simulink model "controllo_SS2023b"  (R2023b)
settings: Solver=VariableStepAuto  StartTime=0.0  StopTime=y1(end,1)  RelTol=1e-3
values from neighbouring files (symbols this model uses):
  A_ob = A - L_kf*C    [LQ_KF.m]    (also in LQ_KF_version1.m; LQ_KF_version2.m; LQ_Luenberger.m = A - L*C; LQ_prova.m)
  B_ob = [ B - L_kf*D, L_kf]    [LQ_KF.m]    (also in LQ_KF_version1.m; LQ_KF_version2.m; LQ_Luenberger.m = [ B - L*D, L]; LQ_prova.m)
  C_ob = eye(n)    [LQ_KF.m]    (also in LQ_KF_version1.m; LQ_KF_version2.m; LQ_Luenberger.m; LQ_prova.m)
  D_ob = zeros(n, m+p)    [LQ_KF.m]    (also in LQ_KF_version1.m; LQ_KF_version2.m; LQ_Luenberger.m; LQ_prova.m)
  Ken_eta = K(:, 4)    [LQ_KF.m]    (also in LQ_KF_version1.m; LQ_KF_version2.m = Ken(:, n+1:end); LQ_Luenberger.m; LQ_prova.m = Ken(:, n+1:end))
  Ken_x = K(:, 1:3)    [LQ_KF.m]    (also in LQ_KF_version1.m; LQ_KF_version2.m = Ken(:, 1:n); LQ_Luenberger.m; LQ_prova.m = Ken(:, 1:n))
undefined symbols (not defined in the file or in its folder): Lc, Rtot, x1_eq0, x2_eq0, x3_eq0
libraries: simulink x1
settings Model: Creator=Pronto all'uso  LastModifiedBy=Pronto all'uso

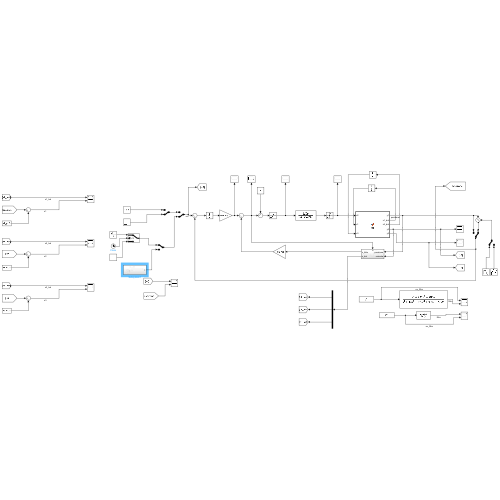
[thumbnail: Simulink's stored preview of the top-level diagram]
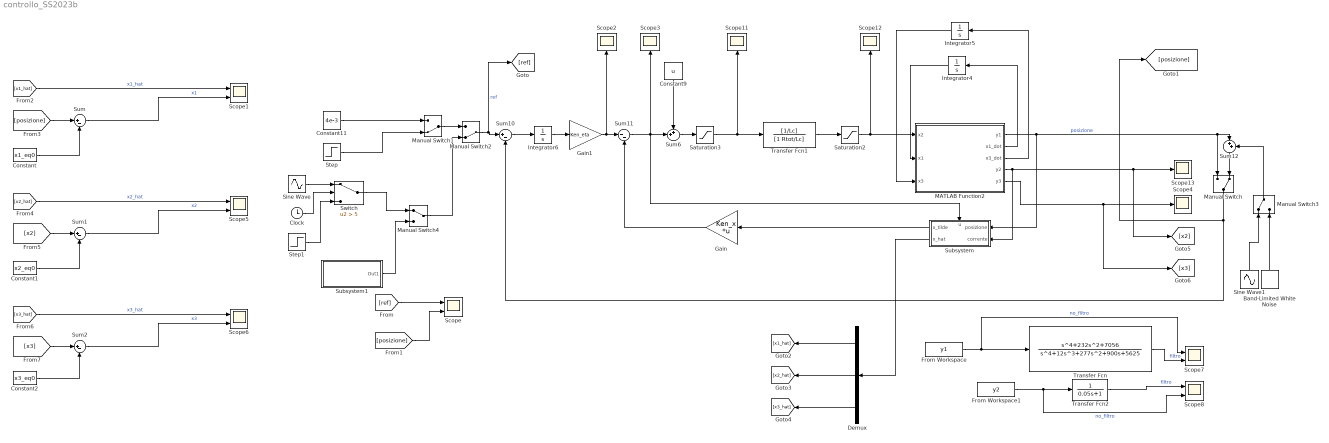
== system controllo_SS2023b ==
  Band-Limited White Noise : simulink/Sources/Band-Limited White Noise  Cov=[8.9934e-8*0.002]  Ts=0.002  seed=[23341]
  Clock : Clock
  Constant : Constant  Value=x1_eq0
  Constant1 : Constant  Value=x2_eq0
  Constant11 : Constant  Value=4e-3
  Constant2 : Constant  Value=x3_eq0
  Constant9 : Constant  Value=u
  Demux : Demux  Outputs=3
  From Workspace : FromWorkspace  VariableName=y1
  From Workspace1 : FromWorkspace  VariableName=y2
  Gain : Gain  Gain=Ken_x  Multiplication=Matrix(K*u) (u vector)
  Gain1 : Gain  Gain=Ken_eta
  Integrator4 : Integrator
  Integrator5 : Integrator
  Integrator6 : Integrator
  MATLAB Function2 : MATLAB Function  TreatAsAtomicUnit=on
  Manual Switch : ManualSwitch  CurrentSetting=0
  Manual Switch1 : ManualSwitch  CurrentSetting=0
  Manual Switch2 : ManualSwitch  CurrentSetting=0
  Manual Switch3 : ManualSwitch
  Manual Switch4 : ManualSwitch
  Saturation2 : Saturate  UpperLimit=3  LowerLimit=0
  Saturation3 : Saturate  UpperLimit=24  LowerLimit=0
  Scope{,1,5..8} (6 alike) : Scope  NumInputPorts=2
  Scope{2..4,11..13} (6 alike) : Scope
  Sine Wave : Sin  Amplitude=0.0005  Bias=0.004  SampleTime=0
  Sine Wave1 : Sin  Amplitude=0.00001  Frequency=50  SampleTime=0.002
  Step : Step  Time=2  After=0.003  SampleTime=0.002
  Step1 : Step  Time=3  After=0.004  SampleTime=0
  Subsystem : Subsystem
      settings: PortSchema="{\"entries\":[{\"content\":{\"sides\":[{\"content\":{\"connectorIds\":[\"In1\",\"In2\"]},\"type\":\"ConnectorPlacement.EquallySpacedRectSide\",\"uuid\":\"698df1f3-7755-43c0-a5fb-5bdaf8e9b8ef\"},{\"content\":{\"connectorIds\":[\"Out1\",\"Out2\"],\"side\":\"RIGHT\"},\"type\":\"ConnectorPlacement.EquallySpacedRectSide\",\"uuid\":\"f0019f40-b27c-431f-9c37-04fd54da4bcb\"},{\"content\":{\"connectorIds\":[\"In3\"],\"side\":\"TOP\"},\"type\":\"ConnectorPlacement.EquallySpacedRectSide\",\"uuid\":\"7983fe5a-f7de-4e42-be2b-50e780fdde63\"}]},\"type\":\"ConnectorPlacement.EquallySpacedConnector\",\"uuid\":\"65d76084-d1f3-463d-b10f-a9e5fd5bbc83\"}],\"packageUris\":[\"http://schema.mathworks.com/mf0/Connector/R2020b\"],\"version\":\"1.0\"}"
  Subsystem1 : Subsystem
  Sum{,1..2,10} (4 alike) : Sum  Inputs=|+-
  Sum11 : Sum  Inputs=|--
  Sum12 : Sum  Inputs=|++
  Sum6 : Sum  Inputs=++|
  Switch : Switch  Criteria=u2 > Threshold  Threshold=5  SaturateOnIntegerOverflow=off  InputSameDT=off
  Transfer Fcn : TransferFcn  Numerator=[1 0 232 0 7056]  Denominator=[1 12 277 900 5625]
  Transfer Fcn1 : TransferFcn  Numerator=[1/Lc]  Denominator=[1 Rtot/Lc]
  Transfer Fcn2 : TransferFcn  Denominator=[0.05 1]
  wires:
  Constant9/1 -> Sum6/1
  [posizione] -> Scope/2
  [ref] -> Scope/1
  MATLAB Function2/4(y2) -> [x2], Scope13/1, Subsystem/2(corrente)
  Sum10/1 -> Integrator6/1
  Step/1 -> Manual Switch1/2
  Saturation3/1 -> Transfer Fcn1/1, Scope11/1
  Manual Switch/1 -> [posizione], Sum10/2
  Constant11/1 -> Manual Switch1/1
  MATLAB Function2/5(y3) -> [x3], Scope4/1
  MATLAB Function2/1(y1) -> Sum12/1, Manual Switch/1, Subsystem/1(posizione)  "posizione"
  MATLAB Function2/2(x1_dot) -> Integrator4/1
  Sum12/1 -> Manual Switch/2
  Integrator4/1 -> MATLAB Function2/2(x1)
  Band-Limited White Noise/1 -> Manual Switch3/2
  Sum6/1 -> Saturation3/1
  Manual Switch2/1 -> [ref], Sum10/1  "ref"
  Integrator6/1 -> Gain1/1
  Sine Wave1/1 -> Manual Switch3/1
  Manual Switch3/1 -> Sum12/2
  Integrator5/1 -> MATLAB Function2/3(x3)
  Saturation2/1 -> MATLAB Function2/1(x2), Scope12/1
  Gain1/1 -> Sum11/1, Scope2/1
  Sum11/1 -> Subsystem/3(u), Scope3/1, Sum6/2
  MATLAB Function2/3(x3_dot) -> Integrator5/1
  Transfer Fcn1/1 -> Saturation2/1
  Manual Switch1/1 -> Manual Switch2/1
  Demux/1 -> [x1_hat]
  Demux/2 -> [x2_hat]
  Demux/3 -> [x3_hat]
  Gain/1 -> Sum11/2
  [x1_hat] -> Scope1/1  "x1_hat"
  [posizione] -> Sum/1
  Constant/1 -> Sum/2
  Sum/1 -> Scope1/2  "x1"
  Sum1/1 -> Scope5/2  "x2"
  [x2] -> Sum1/1
  [x2_hat] -> Scope5/1  "x2_hat"
  Constant1/1 -> Sum1/2
  Sum2/1 -> Scope6/2  "x3"
  [x3] -> Sum2/1
  [x3_hat] -> Scope6/1  "x3_hat"
  Constant2/1 -> Sum2/2
  Subsystem/1(x_tilde) -> Gain/1
  Subsystem/2(x_hat) -> Demux/1
  Manual Switch4/1 -> Manual Switch2/2
  Subsystem1/1(Out1) -> Manual Switch4/2
  Sine Wave/1 -> Switch/1
  Switch/1 -> Manual Switch4/1
  Step1/1 -> Switch/3
  Clock/1 -> Switch/2
  From Workspace/1 -> Transfer Fcn/1, Scope7/1  "no_filtro"
  From Workspace1/1 -> Scope8/2, Transfer Fcn2/1  "no_filtro"
  Transfer Fcn2/1 -> Scope8/1  "filtro"
  Transfer Fcn/1 -> Scope7/2  "filtro"

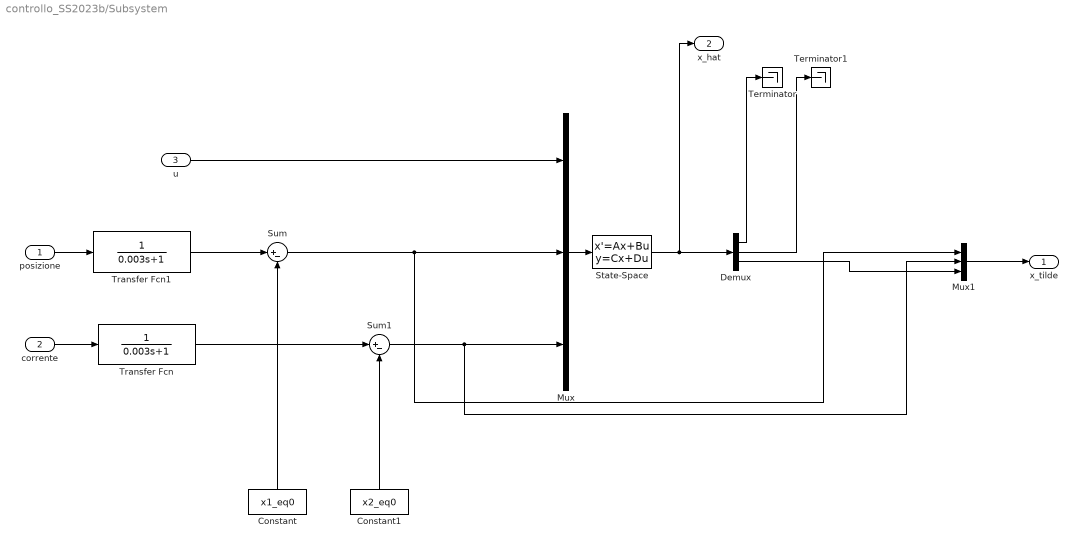
== system controllo_SS2023b/Subsystem ==
  posizione : Inport
  corrente : Inport  Port=2
  u : Inport  Port=3
  Constant : Constant  Value=x1_eq0
  Constant1 : Constant  Value=x2_eq0
  Demux : Demux  Outputs=3
  Mux : Mux  Inputs=3
  Mux1 : Mux  Inputs=3
  State-Space : StateSpace  A=A_ob  B=B_ob  C=C_ob  D=D_ob  InitialCondition=[0, 0, 0]  ParameterTunability=Unconstrained
  Sum : Sum  Inputs=|+-
  Sum1 : Sum  Inputs=|+-
  Terminator : Terminator
  Terminator1 : Terminator
  Transfer Fcn : TransferFcn  Denominator=[0.003 1]
  Transfer Fcn1 : TransferFcn  Denominator=[0.003 1]
  x_tilde : Outport
  x_hat : Outport  Port=2
  wires:
  posizione/1 -> Transfer Fcn1/1
  Constant/1 -> Sum/2
  Constant1/1 -> Sum1/2
  corrente/1 -> Transfer Fcn/1
  u/1 -> Mux/1
  Sum/1 -> Mux1/1, Mux/2
  Sum1/1 -> Mux1/2, Mux/3
  Mux/1 -> State-Space/1
  Mux1/1 -> x_tilde/1
  State-Space/1 -> x_hat/1, Demux/1
  Demux/1 -> Terminator/1
  Demux/2 -> Terminator1/1
  Demux/3 -> Mux1/3
  Transfer Fcn/1 -> Sum1/1
  Transfer Fcn1/1 -> Sum/1

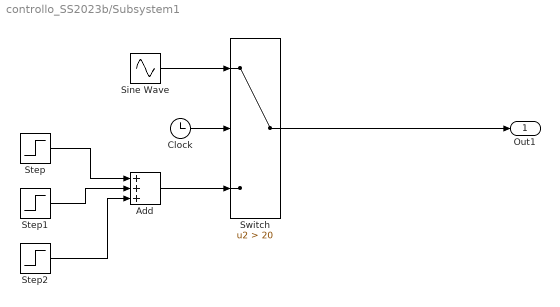
== system controllo_SS2023b/Subsystem1 ==
  Add : Sum  Inputs=+++
  Clock : Clock
  Sine Wave : Sin  Amplitude=0.002  Bias=0.005  SampleTime=0
  Step : Step  Time=3  After=0.003  SampleTime=0
  Step1 : Step  Time=5  After=0.004  SampleTime=0
  Step2 : Step  Time=10  After=-0.002  SampleTime=0
  Switch : Switch  Criteria=u2 > Threshold  Threshold=20  SaturateOnIntegerOverflow=off  InputSameDT=off
  Out1 : Outport
  wires:
  Switch/1 -> Out1/1
  Step/1 -> Add/1
  Step1/1 -> Add/2
  Step2/1 -> Add/3
  Add/1 -> Switch/3
  Clock/1 -> Switch/2
  Sine Wave/1 -> Switch/1

== matlab function controllo_SS2023b/MATLAB Function2 ==
  data: y1 output; x2 input; x1_dot output; x1 input; x3 input; x3_dot output; y2 output; y3 output
function [y1,x1_dot, x3_dot, y2, y3] = fcn(x2, x1, x3)
    m = 0.0657;
    g = 9.81;
    k_mag = 2.4405e-05;
    Rtot = 9.7585;
    Lc = 0.3708;
    y0 = 0.012;
    
    x1_dot = x3;
    x3_dot = (k_mag/m)*(x2/(y0-x1))^2 - g;

    if x1 <= 0 && x3_dot < 0
        x1 = 0;
        x3 = 0;
        x3_dot = 0;
    end
y1 = x1;
y2 = x2;
y3 = x3;
